simulink model "quickTest"  (R2018a)
settings: Solver=ode4  StartTime=0.0  StopTime=4  FixedStep=Ts  RelTol=1e-3
undefined symbols (not defined in the file or in its folder): ground_W, ground_WN
settings Model: Creator=nicola  LastModifiedBy=nicola

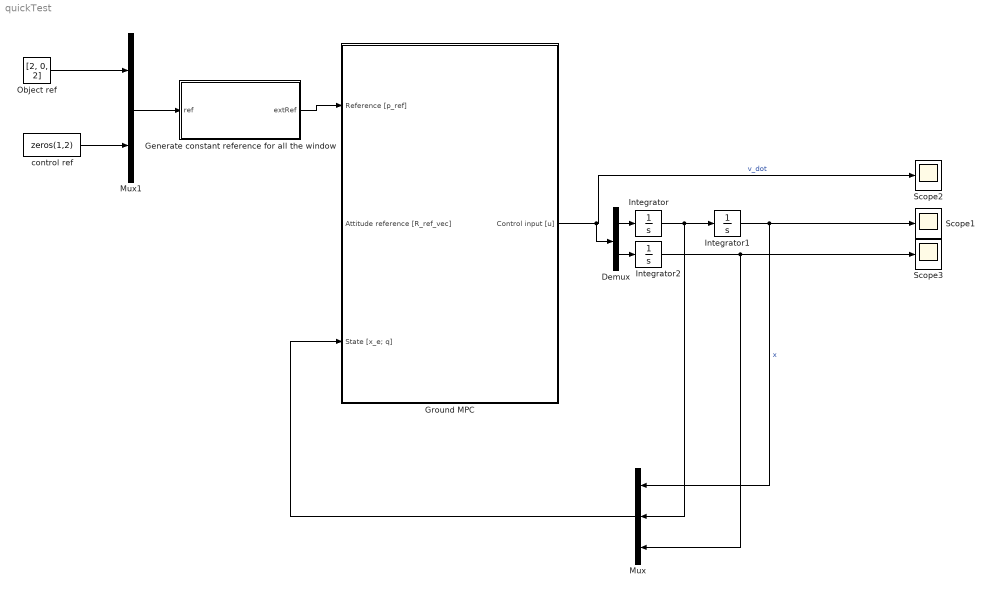
== system quickTest ==
  Demux : Demux  Outputs=2
  Generate constant reference for all the window : MATLAB Function  TreatAsAtomicUnit=on
  Ground MPC : Subsystem
  Integrator : Integrator
  Integrator1 : Integrator
  Integrator2 : Integrator
  Mux : Mux  Inputs=3
  Mux1 : Mux  Inputs=2
  Object ref : Constant  Value=[2, 0, 2]
  Scope1 : Scope
  Scope2 : Scope
  Scope3 : Scope
  control ref : Constant  Value=zeros(1,2)
  wires:
  control ref/1 -> Mux1/2
  Mux1/1 -> Generate constant reference for all the window/1(ref)
  Mux/1 -> Ground MPC/3(State [x_e; q])
  Object ref/1 -> Mux1/1
  Generate constant reference for all the window/1(extRef) -> Ground MPC/1(Reference [p_ref])
  Ground MPC/1("Control input [u] ") -> Scope2/1, Demux/1  "v_dot"
  Integrator1/1 -> Mux/1, Scope1/1  "x"
  Integrator/1 -> Integrator1/1, Mux/2
  Demux/1 -> Integrator/1
  Demux/2 -> Integrator2/1
  Integrator2/1 -> Mux/3, Scope3/1

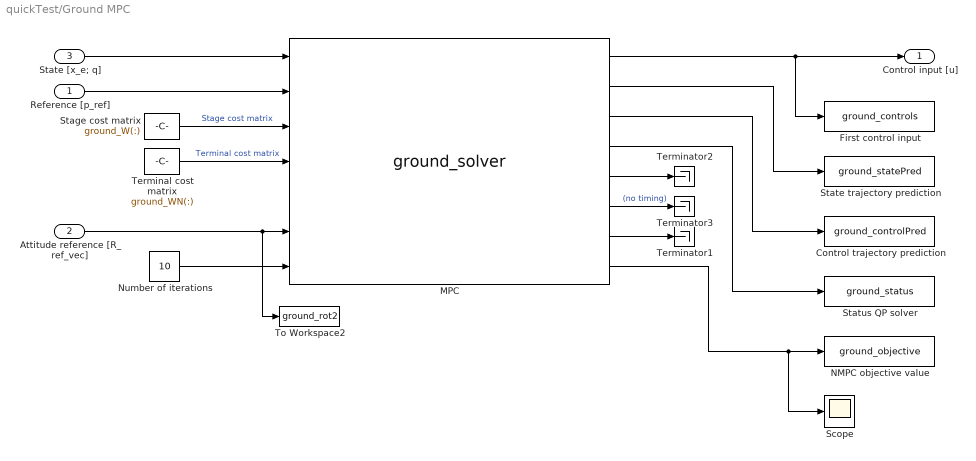
== system quickTest/Ground MPC ==
  Reference [p_ref] : Inport
  Attitude reference [R_ref_vec] : Inport  Port=2
  State [x_e; q] : Inport  Port=3
  Control trajectory prediction : ToWorkspace  VariableName=ground_controlPred  SaveFormat=Structure With Time  SampleTime=-1
  First control input : ToWorkspace  VariableName=ground_controls  SaveFormat=Structure With Time  SampleTime=-1
  MPC : S-Function  FunctionName=ground_solver  Parameters=ground_xInit, ground_zInit, ground_uInit, ground_W, ground_WN, ground_bValues  SFunctionDeploymentMode=off  EnableBusSupport=off  mask(Legacy Function){SFunctionSpec=acado_step(ACADOinput u1[1], ACADOoutput y1[1]), ShowSpec=off}
      mask prompts: ShowSpec "Display function specification"
      mask help:
      | This block allows you to call the legacy functions specified by the following Legacy Code Tool definition:
      | def.SFunctionName = 'acado_solver_sfun';
      | def.OutputFcnSpec = 'acado_step(ACADOinput u1[1], ACADOoutput y1[1])';
      | def.StartFcnSpec = 'acado_initialize( void )';
      | def.TerminateFcnSpec = 'acado_cleanup( void )';
      | def.HeaderFiles = {'acado_common.h', 'acado_solver_sfunction.h'};
      | def.SourceFiles = {'acado_solver.c', 'acado_integrator.c', 'acado_auxiliary_functions.c', 'acado_solver_sfunction.c', 'acado_qpoases_interface.cpp', 'qpoases/SRC/Bounds.cpp', 'qpoases/SRC/Constraints.cpp', 'qpoases/SRC/CyclingManager.cpp', 'qpoases/SRC/Indexlist.cpp', 'qpoases/SRC/MessageHandling.cpp', 'qpoases/SRC/QProblem.cpp', 'qpoases/SRC/QProblemB.cpp', 'qpoases/SRC/SubjectTo.cpp', 'qpoases/SRC/Utils.cpp', 'qpoases/SRC/EXTRAS/SolutionAnalysis.cpp'};
      | def.IncPaths = {'qpoases', 'qpoases/INCLUDE', 'qpoases/SRC'};
      | def.Options.language = 'C++';
      mask Help: <p>This block was generated automatically by the Legacy Code Tool. For detailed help on this tool, call<a href="matlab:legacy_code('help')"> legacy_code('help')</a>.</p>
      mask Callback ShowSpec:
      | if strcmp(get_param(gcbh, 'ShowSpec'), 'on')
      |   set_param(gcbh, 'MaskDisplay', sprintf('fprintf(''%s'');', get_param(gcbh, 'SFunctionSpec')));
      | else
      |   set_param(gcbh, 'MaskDisplay', sprintf('fprintf(''%s'');', get_param(gcbh, 'FunctionName')));
      | end
      mask Display: fprintf('ground_solver');
  NMPC objective value : ToWorkspace  VariableName=ground_objective  SaveFormat=Structure With Time  SampleTime=-1
  Number of iterations : Constant  Value=10  OutDataTypeStr=double
  Scope : Scope
  Stage cost matrix : Constant  Value=ground_W(:)  OutDataTypeStr=double
  State trajectory prediction : ToWorkspace  VariableName=ground_statePred  SaveFormat=Structure With Time  SampleTime=-1
  Status QP solver : ToWorkspace  VariableName=ground_status  SaveFormat=Structure With Time  SampleTime=-1
  Terminal cost matrix : Constant  Value=ground_WN(:)  OutDataTypeStr=double
  Terminator1 : Terminator
  Terminator2 : Terminator
  Terminator3 : Terminator
  To Workspace2 : ToWorkspace  VariableName=ground_rot2  SampleTime=-1
  "Control input [u] " : Outport
  wires:
  MPC/3 -> Control trajectory prediction/1
  MPC/7 -> Terminator1/1
  Stage cost matrix/1 -> MPC/3  "Stage cost matrix"
  MPC/4 -> Status QP solver/1
  MPC/5 -> Terminator2/1
  MPC/1 -> "Control input [u] "/1, First control input/1
  Number of iterations/1 -> MPC/7
  MPC/8 -> Scope/1, NMPC objective value/1
  Terminal cost matrix/1 -> MPC/4  "Terminal cost matrix"
  MPC/2 -> State trajectory prediction/1
  MPC/6 -> Terminator3/1  "(no timing)"
  State [x_e; q]/1 -> MPC/1
  Reference [p_ref]/1 -> MPC/2
  Attitude reference [R_ref_vec]/1 -> To Workspace2/1, MPC/6

== matlab function quickTest/Generate constant reference for all the window ==
  data: ref input double; extRef output
function extRef = constReference (ref)
    % Need to be hardcoded each time
    N = 10;
    
    ref = reshape (ref,length(ref),1);
    yN = ref(1:end-2);
    y = [repmat(ref',N,1)].';
    extRef = [y(:);yN];
end
